simulink model "PTC_MBDS_StringMid_Sample"  (R2013a)
settings: Solver=FixedStepDiscrete  StartTime=0.0  StopTime=100  FixedStep=0.02  RelTol=1e-3
undefined symbols (not defined in the file): PTC_MBDS_MaxStringLength_Fcn
libraries: PTC_MBDS_LIB x20, simulink_extras x1
settings Model: Creator=uidl7367  LastModifiedBy=sundeep.tuteja
settings DataIOCC: SignalLoggingSaveFormat=ModelDataLogs
settings OptimizationCC: ExpressionDepthLimit=2147483647  InitFltsAndDblsToZero=on
settings DebuggingCC: SaveWithParameterizedLinksMsg=none  SignalResolutionControl=TryResolveAllWithWarning  InheritedTsInSrcMsg=none  MultiTaskDSMMsg=warning  MultiTaskCondExecSysMsg=none  FcnCallInpInsideContextMsg=UseLocalSettings  StrictBusMsg=Warning
settings RTWCC: IncludeERTFirstTime=on
settings GRTTargetCC: TargetFcnLib=ansi_tfl_tmw.mat  CombineOutputUpdateFcns=off  GRTInterface=on

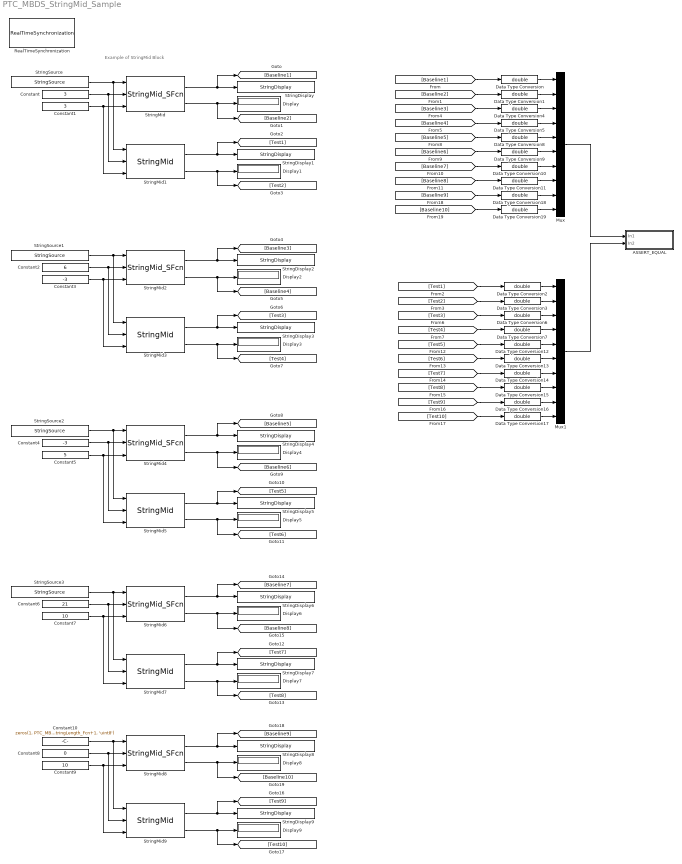
== system PTC_MBDS_StringMid_Sample ==
  note: Example of StringMid Block
  ASSERT_EQUAL : Subsystem
  Constant : Constant  InitFcn=|  Value=3  VectorParams1D=off  OutDataTypeStr=int16
      | if(exist('MBDS_BlockCallback', 'file'))
      |    MBDS_BlockCallback('Update', gcb);  
      | end
  Constant1 : Constant  InitFcn=|  Value=3  VectorParams1D=off  OutDataTypeStr=int8
      | if(exist('MBDS_BlockCallback', 'file'))
      |    MBDS_BlockCallback('Update', gcb);  
      | end
  Constant10 : Constant  InitFcn=|  Value=zeros(1, PTC_MBDS_MaxStringLength_Fcn+1, 'uint8')  VectorParams1D=off
      | if(exist('MBDS_BlockCallback', 'file'))
      |    MBDS_BlockCallback('Update', gcb);  
      | end
  Constant2 : Constant  InitFcn=|  Value=6  VectorParams1D=off  OutDataTypeStr=int16
      | if(exist('MBDS_BlockCallback', 'file'))
      |    MBDS_BlockCallback('Update', gcb);  
      | end
  Constant3 : Constant  InitFcn=|  Value=-3  VectorParams1D=off  OutDataTypeStr=int8
      | if(exist('MBDS_BlockCallback', 'file'))
      |    MBDS_BlockCallback('Update', gcb);  
      | end
  Constant4 : Constant  InitFcn=|  Value=-3  VectorParams1D=off  OutDataTypeStr=int16
      | if(exist('MBDS_BlockCallback', 'file'))
      |    MBDS_BlockCallback('Update', gcb);  
      | end
  Constant5 : Constant  InitFcn=|  Value=5  VectorParams1D=off  OutDataTypeStr=int8
      | if(exist('MBDS_BlockCallback', 'file'))
      |    MBDS_BlockCallback('Update', gcb);  
      | end
  Constant6 : Constant  InitFcn=|  Value=21  VectorParams1D=off  OutDataTypeStr=int16
      | if(exist('MBDS_BlockCallback', 'file'))
      |    MBDS_BlockCallback('Update', gcb);  
      | end
  Constant7 : Constant  InitFcn=|  Value=10  VectorParams1D=off  OutDataTypeStr=int8
      | if(exist('MBDS_BlockCallback', 'file'))
      |    MBDS_BlockCallback('Update', gcb);  
      | end
  Constant8 : Constant  InitFcn=|  Value=0  VectorParams1D=off  OutDataTypeStr=int16
      | if(exist('MBDS_BlockCallback', 'file'))
      |    MBDS_BlockCallback('Update', gcb);  
      | end
  Constant9 : Constant  InitFcn=|  Value=10  VectorParams1D=off  OutDataTypeStr=int8
      | if(exist('MBDS_BlockCallback', 'file'))
      |    MBDS_BlockCallback('Update', gcb);  
      | end
  Data Type Conversion{,1..19} (20 alike) : DataTypeConversion  OutDataTypeStr=double  SaturateOnIntegerOverflow=on
  Display{,1..9} (10 alike) : Display
  Mux : Mux  Inputs=10
  Mux1 : Mux  Inputs=10
  RealTimeSynchronization : PTC_MBDS_LIB/MBDS Standard Library/Extended Operations/HMI/RealTimeSynchronization  Enable=off  PTC_MBDS_BlockVersion=5.32  PTC_BlockType=PTC_MBDS_RealTimeSynchronization
  StringDisplay : PTC_MBDS_LIB/MBDS Standard Library/Extended Operations/String Operations/StringDisplay  MaxRowCount=1  BlockSignature=----------  PTC_MBDS_BlockVersion=5.32  PTC_BlockType=PTC_MBDS_StringDisplay  DisplayString=cde  MaxStringLength=PTC_MBDS_MaxStringLength_Fcn
  StringDisplay1 : PTC_MBDS_LIB/MBDS Standard Library/Extended Operations/String Operations/StringDisplay  MaxRowCount=1  BlockSignature=----------  PTC_MBDS_BlockVersion=5.32  PTC_BlockType=PTC_MBDS_StringDisplay  DisplayString=cde  MaxStringLength=PTC_MBDS_MaxStringLength_Fcn
  StringDisplay2 : PTC_MBDS_LIB/MBDS Standard Library/Extended Operations/String Operations/StringDisplay  MaxRowCount=1  BlockSignature=----------  PTC_MBDS_BlockVersion=5.32  PTC_BlockType=PTC_MBDS_StringDisplay  DisplayString=ab  MaxStringLength=PTC_MBDS_MaxStringLength_Fcn
  StringDisplay3 : PTC_MBDS_LIB/MBDS Standard Library/Extended Operations/String Operations/StringDisplay  MaxRowCount=1  BlockSignature=----------  PTC_MBDS_BlockVersion=5.32  PTC_BlockType=PTC_MBDS_StringDisplay  DisplayString=ab  MaxStringLength=PTC_MBDS_MaxStringLength_Fcn
  StringDisplay4 : PTC_MBDS_LIB/MBDS Standard Library/Extended Operations/String Operations/StringDisplay  MaxRowCount=1  BlockSignature=----------  PTC_MBDS_BlockVersion=5.32  PTC_BlockType=PTC_MBDS_StringDisplay  DisplayString=bcd  MaxStringLength=PTC_MBDS_MaxStringLength_Fcn
  StringDisplay5 : PTC_MBDS_LIB/MBDS Standard Library/Extended Operations/String Operations/StringDisplay  MaxRowCount=1  BlockSignature=----------  PTC_MBDS_BlockVersion=5.32  PTC_BlockType=PTC_MBDS_StringDisplay  DisplayString=bcd  MaxStringLength=PTC_MBDS_MaxStringLength_Fcn
  StringDisplay6 : PTC_MBDS_LIB/MBDS Standard Library/Extended Operations/String Operations/StringDisplay  MaxRowCount=1  BlockSignature=----------  PTC_MBDS_BlockVersion=5.32  PTC_BlockType=PTC_MBDS_StringDisplay  DisplayString=oHfzghXsM8BRVBPg6lqYE  MaxStringLength=PTC_MBDS_MaxStringLength_Fcn
  StringDisplay7 : PTC_MBDS_LIB/MBDS Standard Library/Extended Operations/String Operations/StringDisplay  MaxRowCount=1  BlockSignature=----------  PTC_MBDS_BlockVersion=5.32  PTC_BlockType=PTC_MBDS_StringDisplay  DisplayString=oHfzghXsM8BRVBPg6lqYE  MaxStringLength=PTC_MBDS_MaxStringLength_Fcn
  StringDisplay8 : PTC_MBDS_LIB/MBDS Standard Library/Extended Operations/String Operations/StringDisplay  MaxRowCount=1  BlockSignature=----------  PTC_MBDS_BlockVersion=5.32  PTC_BlockType=PTC_MBDS_StringDisplay  MaxStringLength=PTC_MBDS_MaxStringLength_Fcn
  StringDisplay9 : PTC_MBDS_LIB/MBDS Standard Library/Extended Operations/String Operations/StringDisplay  MaxRowCount=1  BlockSignature=----------  PTC_MBDS_BlockVersion=5.32  PTC_BlockType=PTC_MBDS_StringDisplay  MaxStringLength=PTC_MBDS_MaxStringLength_Fcn
  StringMid : S-Function  InitFcn=|  FunctionName=StringMid_SFcn  Parameters=boolean(ENO_Enabled), uint16(MaxStringLength)  EnableBusSupport=off  mask(StringMid){MBDS_LibraryBlock=on, ENO_Enabled=on, MBDS_BlockVersion=05.40}
      | if(exist('MBDS_BlockCallback', 'file'))
      |    MBDS_BlockCallback('Update', gcb);
      | end
      mask prompts: MBDS_LibraryBlock "MBDS Library Block"; ENO_Enabled "Show ENO port"; MBDS_BlockVersion "Block version:"
      mask help: Extracts the middle part of a string at input port In. The substring position is specified by the input port P and the substring length is given by input port L.
      mask init:
      | MBDS_BlockCallback('Copy', gcb);
      | MaxStringLength = 1 + GetStringLen();
      | maskdisplay = ['disp(''Mid'')' 10];
      | maskdisplay = [maskdisplay 'port_label(''input'', 1, ''In'')' 10];
      | maskdisplay = [maskdisplay 'port_label(''input'', 2, ''L'')' 10];
      | maskdisplay = [maskdisplay 'port_label(''input'', 3, ''P'')' 10];
      | maskdisplay = [maskdisplay 'port_label(''output'', 1, ''Out'')' 10];
      | if(ENO_Enabled)
      |    maskdisplay = [maskdisplay 'port_label(''output'', 2, ''ENO'')' 10];
      | end
      | set_param(gcbh, 'maskdisplay', maskdisplay)
      mask Help: eval(['open([workdir(''Library_Dir:''),''\Blockset\Help\'',get_param(gcb,''MaskType''),''.html''])'])
      mask Display:
      | disp('Mid')
      | port_label('input', 1, 'In')
      | port_label('input', 2, 'L')
      | port_label('input', 3, 'P')
      | port_label('output', 1, 'Out')
      | port_label('output', 2, 'ENO')
  StringMid{1,3,5,7,9} (5 alike) : PTC_MBDS_LIB/MBDS Standard Library/Extended Operations/String Operations/StringMid  ENO_Enabled=on  MaxStringLength=PTC_MBDS_MaxStringLength_Fcn  PTC_MBDS_BlockVersion=5.32  PTC_BlockType=PTC_MBDS_StringMid
  StringMid2 : S-Function  InitFcn=|  FunctionName=StringMid_SFcn  Parameters=boolean(ENO_Enabled), uint16(MaxStringLength)  EnableBusSupport=off  mask(StringMid){MBDS_LibraryBlock=on, ENO_Enabled=on, MBDS_BlockVersion=05.40}
      | if(exist('MBDS_BlockCallback', 'file'))
      |    MBDS_BlockCallback('Update', gcb);
      | end
      mask prompts: MBDS_LibraryBlock "MBDS Library Block"; ENO_Enabled "Show ENO port"; MBDS_BlockVersion "Block version:"
      mask help: Extracts the middle part of a string at input port In. The substring position is specified by the input port P and the substring length is given by input port L.
      mask init: same as PTC_MBDS_StringMid_Sample/StringMid
      mask Help: eval(['open([workdir(''Library_Dir:''),''\Blockset\Help\'',get_param(gcb,''MaskType''),''.html''])'])
      mask Display:
      | disp('Mid')
      | port_label('input', 1, 'In')
      | port_label('input', 2, 'L')
      | port_label('input', 3, 'P')
      | port_label('output', 1, 'Out')
      | port_label('output', 2, 'ENO')
  StringMid4 : S-Function  InitFcn=|  FunctionName=StringMid_SFcn  Parameters=boolean(ENO_Enabled), uint16(MaxStringLength)  EnableBusSupport=off  mask(StringMid){MBDS_LibraryBlock=on, ENO_Enabled=on, MBDS_BlockVersion=05.40}
      | if(exist('MBDS_BlockCallback', 'file'))
      |    MBDS_BlockCallback('Update', gcb);
      | end
      mask prompts: MBDS_LibraryBlock "MBDS Library Block"; ENO_Enabled "Show ENO port"; MBDS_BlockVersion "Block version:"
      mask help: Extracts the middle part of a string at input port In. The substring position is specified by the input port P and the substring length is given by input port L.
      mask init: same as PTC_MBDS_StringMid_Sample/StringMid
      mask Help: eval(['open([workdir(''Library_Dir:''),''\Blockset\Help\'',get_param(gcb,''MaskType''),''.html''])'])
      mask Display:
      | disp('Mid')
      | port_label('input', 1, 'In')
      | port_label('input', 2, 'L')
      | port_label('input', 3, 'P')
      | port_label('output', 1, 'Out')
      | port_label('output', 2, 'ENO')
  StringMid6 : S-Function  InitFcn=|  FunctionName=StringMid_SFcn  Parameters=boolean(ENO_Enabled), uint16(MaxStringLength)  EnableBusSupport=off  mask(StringMid){MBDS_LibraryBlock=on, ENO_Enabled=on, MBDS_BlockVersion=05.40}
      | if(exist('MBDS_BlockCallback', 'file'))
      |    MBDS_BlockCallback('Update', gcb);
      | end
      mask prompts: MBDS_LibraryBlock "MBDS Library Block"; ENO_Enabled "Show ENO port"; MBDS_BlockVersion "Block version:"
      mask help: Extracts the middle part of a string at input port In. The substring position is specified by the input port P and the substring length is given by input port L.
      mask init: same as PTC_MBDS_StringMid_Sample/StringMid
      mask Help: eval(['open([workdir(''Library_Dir:''),''\Blockset\Help\'',get_param(gcb,''MaskType''),''.html''])'])
      mask Display:
      | disp('Mid')
      | port_label('input', 1, 'In')
      | port_label('input', 2, 'L')
      | port_label('input', 3, 'P')
      | port_label('output', 1, 'Out')
      | port_label('output', 2, 'ENO')
  StringMid8 : S-Function  InitFcn=|  FunctionName=StringMid_SFcn  Parameters=boolean(ENO_Enabled), uint16(MaxStringLength)  EnableBusSupport=off  mask(StringMid){MBDS_LibraryBlock=on, ENO_Enabled=on, MBDS_BlockVersion=05.40}
      | if(exist('MBDS_BlockCallback', 'file'))
      |    MBDS_BlockCallback('Update', gcb);
      | end
      mask prompts: MBDS_LibraryBlock "MBDS Library Block"; ENO_Enabled "Show ENO port"; MBDS_BlockVersion "Block version:"
      mask help: Extracts the middle part of a string at input port In. The substring position is specified by the input port P and the substring length is given by input port L.
      mask init: same as PTC_MBDS_StringMid_Sample/StringMid
      mask Help: eval(['open([workdir(''Library_Dir:''),''\Blockset\Help\'',get_param(gcb,''MaskType''),''.html''])'])
      mask Display:
      | disp('Mid')
      | port_label('input', 1, 'In')
      | port_label('input', 2, 'L')
      | port_label('input', 3, 'P')
      | port_label('output', 1, 'Out')
      | port_label('output', 2, 'ENO')
  StringSource : PTC_MBDS_LIB/MBDS Standard Library/Extended Operations/String Operations/StringSource  InputValue=abcdefg  PTC_MBDS_BlockVersion=5.32  PTC_BlockType=PTC_MBDS_StringSource  Value=uint8([97; 98; 99; 100; 101; 102; 103; 0; 0; 0; 0; 0; 0; 0; 0; 0; 0; 0; 0; 0; 0; 0; 0; 0; 0; 0; 0; 0; 0; 0; 0; 0; 0; 0; 0; 0; 0; 0; 0; 0; 0])  MaxStringLength=PTC_MBDS_MaxStringLength_Fcn
  StringSource1 : PTC_MBDS_LIB/MBDS Standard Library/Extended Operations/String Operations/StringSource  InputValue=abcdefg  PTC_MBDS_BlockVersion=5.32  PTC_BlockType=PTC_MBDS_StringSource  Value=uint8([97; 98; 99; 100; 101; 102; 103; 0; 0; 0; 0; 0; 0; 0; 0; 0; 0; 0; 0; 0; 0; 0; 0; 0; 0; 0; 0; 0; 0; 0; 0; 0; 0; 0; 0; 0; 0; 0; 0; 0; 0])  MaxStringLength=PTC_MBDS_MaxStringLength_Fcn
  StringSource2 : PTC_MBDS_LIB/MBDS Standard Library/Extended Operations/String Operations/StringSource  InputValue=abcdefg  PTC_MBDS_BlockVersion=5.32  PTC_BlockType=PTC_MBDS_StringSource  Value=uint8([97; 98; 99; 100; 101; 102; 103; 0; 0; 0; 0; 0; 0; 0; 0; 0; 0; 0; 0; 0; 0; 0; 0; 0; 0; 0; 0; 0; 0; 0; 0; 0; 0; 0; 0; 0; 0; 0; 0; 0; 0])  MaxStringLength=PTC_MBDS_MaxStringLength_Fcn
  StringSource3 : PTC_MBDS_LIB/MBDS Standard Library/Extended Operations/String Operations/StringSource  InputValue=yIoOEjXgsoHfzghXsM8BRVBPg6lqYE  PTC_MBDS_BlockVersion=5.32  PTC_BlockType=PTC_MBDS_StringSource  Value=uint8([121; 73; 111; 79; 69; 106; 88; 103; 115; 111; 72; 102; 122; 103; 104; 88; 115; 77; 56; 66; 82; 86; 66; 80; 103; 54; 108; 113; 89; 69; 0; 0; 0; 0; 0; 0; 0; 0; 0; 0; 0])  MaxStringLength=PTC_MBDS_MaxStringLength_Fcn
  wires:
  Mux/1 -> ASSERT_EQUAL/1(In1)
  Mux1/1 -> ASSERT_EQUAL/2(In2)
  StringSource/1 -> StringMid/1, StringMid1/1
  Constant1/1 -> StringMid/3, StringMid1/3
  Constant/1 -> StringMid/2, StringMid1/2
  StringMid/1 -> [Baseline1], StringDisplay/1
  StringMid1/1 -> [Test1], StringDisplay1/1
  StringMid/2 -> [Baseline2], Display/1
  StringMid1/2 -> [Test2], Display1/1
  [Baseline1] -> Data Type Conversion/1
  Data Type Conversion/1 -> Mux/1
  [Baseline2] -> Data Type Conversion1/1
  Data Type Conversion1/1 -> Mux/2
  [Test1] -> Data Type Conversion2/1
  Data Type Conversion2/1 -> Mux1/1
  Data Type Conversion3/1 -> Mux1/2
  [Test2] -> Data Type Conversion3/1
  StringSource1/1 -> StringMid2/1, StringMid3/1
  Constant3/1 -> StringMid2/3, StringMid3/3
  Constant2/1 -> StringMid2/2, StringMid3/2
  StringMid2/1 -> [Baseline3], StringDisplay2/1
  StringMid3/1 -> [Test3], StringDisplay3/1
  StringMid2/2 -> [Baseline4], Display2/1
  StringMid3/2 -> [Test4], Display3/1
  [Baseline3] -> Data Type Conversion4/1
  [Baseline4] -> Data Type Conversion5/1
  Data Type Conversion4/1 -> Mux/3
  Data Type Conversion5/1 -> Mux/4
  [Test3] -> Data Type Conversion6/1
  Data Type Conversion6/1 -> Mux1/3
  Data Type Conversion7/1 -> Mux1/4
  [Test4] -> Data Type Conversion7/1
  StringSource2/1 -> StringMid4/1, StringMid5/1
  Constant5/1 -> StringMid4/3, StringMid5/3
  Constant4/1 -> StringMid4/2, StringMid5/2
  StringMid4/1 -> [Baseline5], StringDisplay4/1
  StringMid5/1 -> [Test5], StringDisplay5/1
  StringMid4/2 -> [Baseline6], Display4/1
  StringMid5/2 -> [Test6], Display5/1
  StringSource3/1 -> StringMid6/1, StringMid7/1
  Constant7/1 -> StringMid6/3, StringMid7/3
  Constant6/1 -> StringMid6/2, StringMid7/2
  StringMid6/1 -> [Baseline7], StringDisplay6/1
  StringMid7/1 -> [Test7], StringDisplay7/1
  StringMid6/2 -> [Baseline8], Display6/1
  StringMid7/2 -> [Test8], Display7/1
  [Baseline5] -> Data Type Conversion8/1
  Data Type Conversion8/1 -> Mux/5
  [Baseline6] -> Data Type Conversion9/1
  Data Type Conversion9/1 -> Mux/6
  [Baseline7] -> Data Type Conversion10/1
  [Baseline8] -> Data Type Conversion11/1
  Data Type Conversion10/1 -> Mux/7
  Data Type Conversion11/1 -> Mux/8
  [Test5] -> Data Type Conversion12/1
  Data Type Conversion12/1 -> Mux1/5
  [Test6] -> Data Type Conversion13/1
  Data Type Conversion13/1 -> Mux1/6
  [Test7] -> Data Type Conversion14/1
  [Test8] -> Data Type Conversion15/1
  Data Type Conversion14/1 -> Mux1/7
  Data Type Conversion15/1 -> Mux1/8
  Constant10/1 -> StringMid8/1, StringMid9/1
  Constant9/1 -> StringMid8/3, StringMid9/3
  Constant8/1 -> StringMid8/2, StringMid9/2
  StringMid8/1 -> [Baseline9], StringDisplay8/1
  StringMid9/1 -> [Test9], StringDisplay9/1
  StringMid8/2 -> [Baseline10], Display8/1
  StringMid9/2 -> [Test10], Display9/1
  [Test9] -> Data Type Conversion16/1
  [Test10] -> Data Type Conversion17/1
  Data Type Conversion16/1 -> Mux1/9
  Data Type Conversion17/1 -> Mux1/10
  [Baseline9] -> Data Type Conversion18/1
  [Baseline10] -> Data Type Conversion19/1
  Data Type Conversion18/1 -> Mux/9
  Data Type Conversion19/1 -> Mux/10

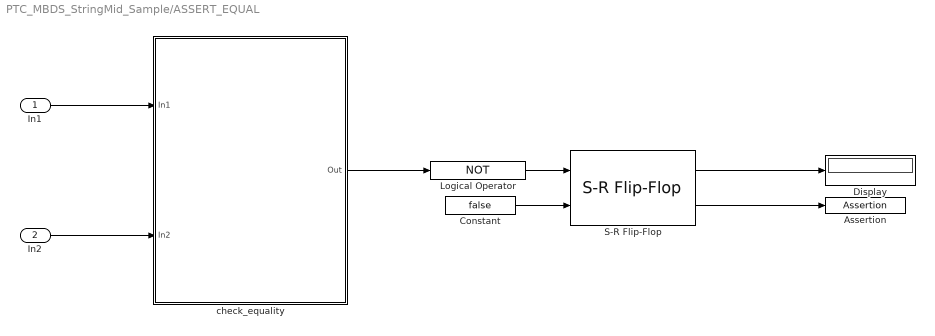
== system PTC_MBDS_StringMid_Sample/ASSERT_EQUAL ==
  In1 : Inport
  In2 : Inport  Port=2
  Assertion : Assertion
  Constant : Constant  Value=false
  Display : Display
  Logical Operator : Logic  Operator=NOT  AllPortsSameDT=off  OutDataTypeStr=boolean
  S-R Flip-Flop : simulink_extras/Flip Flops/S-R Flip-Flop  initial_condition=0
  check_equality : MATLAB Function  TreatAsAtomicUnit=on
  wires:
  S-R Flip-Flop/1 -> Display/1
  check_equality/1(Out) -> Logical Operator/1
  Constant/1 -> S-R Flip-Flop/2
  S-R Flip-Flop/2 -> Assertion/1
  In2/1 -> check_equality/2(In2)
  In1/1 -> check_equality/1(In1)
  Logical Operator/1 -> S-R Flip-Flop/1

== matlab function PTC_MBDS_StringMid_Sample/ASSERT_EQUAL/check_equality ==
  data: In1 input; Out output; In2 input
function Out = check_equality(In1, In2)
%#codegen

Out = isequaln(In1, In2);

end
